simulink model "SortierAlgorithmusVirtuell"  (R2018b)
settings: Solver=FixedStepDiscrete  StartTime=0.0  StopTime=120  RelTol=1e-3  EnableMultiTasking=on
undefined symbols (not defined in the file): sigbuilder_block
libraries: simulink x1, realtime_pacer_lib x1
settings Model: ExtModeTrigDuration=8  Creator=Nici  LastModifiedBy=Nici
settings SolverCC: AutoInsertRateTranBlk=on
settings OptimizationCC: DefaultUnderspecifiedDataType=single  EnhancedBackFolding=on  PassReuseOutputArgsAs=Individual arguments  MaxStackSize=512  OptimizeBlockOrder=speed  DifferentSizesBufferReuse=on  OptimizationCustomize=off
settings DebuggingCC: ParameterTunabilityLossMsg=error  UnderSpecifiedDataTypeMsg=warning
settings HardwareCC: ProdBitPerChar=16  ProdBitPerInt=16  ProdBitPerPointer=32  ProdBitPerSizeT=32  ProdBitPerPtrDiffT=32  ProdLargestAtomicInteger=Integer  ProdLargestAtomicFloat=None  ProdWordSize=16  ProdLongLongMode=on  ProdHWDeviceType=Texas Instruments->C2000
settings SFSimCC: MATLABDynamicMemAlloc=off
settings RTWCC: SystemTargetFile=ert.tlc  HardwareBoard=TI Delfino F2833x  TemplateMakefile=ert_default_tmf  GenerateReport=on  Toolchain=Texas Instruments Code Composer Studio (C2000)  IncludeHyperlinkInReport=on  LaunchReport=on  GenerateTraceInfo=on  GenerateTraceReport=on  GenerateTraceReportSl=on  GenerateTraceReportSf=on  GenerateTraceReportEml=on
settings CodeAppCC: ForceParamTrailComments=on  IgnoreCustomStorageClasses=off  OperatorAnnotations=on  SimulinkDataObjDesc=on  SFDataObjDesc=on  InsertBlockDesc=on
settings ERTTargetCC: CodeReplacementLibrary=TI C28x  SupportContinuousTime=on

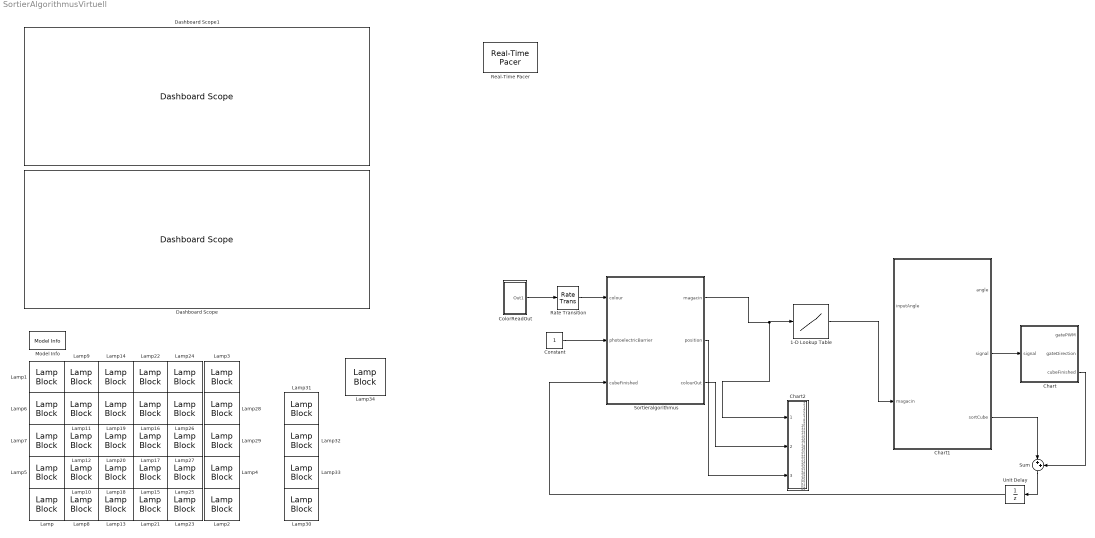
== system SortierAlgorithmusVirtuell ==
  1-D Lookup Table : Lookup_n-D  NumberOfTableDimensions=1  BreakpointsForDimension1=[-1,0,1,2,3,4,5,6]  Table=[-1,-440,-295,-170,-40,85,220,430]  InternalRulePriority=Speed  RndMeth=Simplest  InputSameDT=on
  Chart : Stateflow chart  TreatAsAtomicUnit=on
  Chart1 : Stateflow chart  TreatAsAtomicUnit=on
  Chart2 : Stateflow chart  TreatAsAtomicUnit=on
  ColorReadOut : Subsystem
  Constant : Constant
  Dashboard Scope : DashboardScope  WebBlockId=264  Ymin=-450  Ymax=450
  Dashboard Scope1 : DashboardScope  WebBlockId=268  Ymin=-450  Ymax=450
  Lamp : LampBlock  WebBlockId=196  LabelPosition=Hide
  Lamp1 : LampBlock  WebBlockId=197  LabelPosition=Hide
  Lamp10 : LampBlock  WebBlockId=211  LabelPosition=Hide
  Lamp11 : LampBlock  WebBlockId=212  LabelPosition=Hide
  Lamp12 : LampBlock  WebBlockId=213  LabelPosition=Hide
  Lamp13 : LampBlock  WebBlockId=214  LabelPosition=Hide
  Lamp14 : LampBlock  WebBlockId=215  LabelPosition=Hide
  Lamp15 : LampBlock  WebBlockId=216  LabelPosition=Hide
  Lamp16 : LampBlock  WebBlockId=217  LabelPosition=Hide
  Lamp17 : LampBlock  WebBlockId=218  LabelPosition=Hide
  Lamp18 : LampBlock  WebBlockId=219  LabelPosition=Hide
  Lamp19 : LampBlock  WebBlockId=220  LabelPosition=Hide
  Lamp2 : LampBlock  WebBlockId=249  LabelPosition=Hide
  Lamp20 : LampBlock  WebBlockId=221  LabelPosition=Hide
  Lamp21 : LampBlock  WebBlockId=222  LabelPosition=Hide
  Lamp22 : LampBlock  WebBlockId=223  LabelPosition=Hide
  Lamp23 : LampBlock  WebBlockId=224  LabelPosition=Hide
  Lamp24 : LampBlock  WebBlockId=225  LabelPosition=Hide
  Lamp25 : LampBlock  WebBlockId=226  LabelPosition=Hide
  Lamp26 : LampBlock  WebBlockId=227  LabelPosition=Hide
  Lamp27 : LampBlock  WebBlockId=228  LabelPosition=Hide
  Lamp28 : LampBlock  WebBlockId=252  LabelPosition=Hide
  Lamp29 : LampBlock  WebBlockId=253  LabelPosition=Hide
  Lamp3 : LampBlock  WebBlockId=250  LabelPosition=Hide
  Lamp30 : LampBlock  WebBlockId=257  LabelPosition=Hide
  Lamp31 : LampBlock  WebBlockId=258  LabelPosition=Hide
  Lamp32 : LampBlock  WebBlockId=259  LabelPosition=Hide
  Lamp33 : LampBlock  WebBlockId=260  LabelPosition=Hide
  Lamp34 : LampBlock  WebBlockId=266
  Lamp4 : LampBlock  WebBlockId=251  LabelPosition=Hide
  Lamp5 : LampBlock  WebBlockId=206  LabelPosition=Hide
  Lamp6 : LampBlock  WebBlockId=207  LabelPosition=Hide
  Lamp7 : LampBlock  WebBlockId=208  LabelPosition=Hide
  Lamp8 : LampBlock  WebBlockId=209  LabelPosition=Hide
  Lamp9 : LampBlock  WebBlockId=210  LabelPosition=Hide
  Model Info : simulink/Model-Wide Utilities/Model Info  Frame=on  DisplayStringWithTags=Magazin  HorizontalTextAlignment=Center  LeftAlignmentValue=0.5
  Rate Transition : RateTransition  InitialCondition=1  OutPortSampleTime=0.01
  Real-Time Pacer : realtime_pacer_lib/Real-Time Pacer  simTimePerRealTime=2
  Sortieralgorithmus : Stateflow chart  TreatAsAtomicUnit=on
  Sum : Sum  Inputs=|++
  Unit Delay : UnitDelay  SampleTime=-1
  wires:
  1-D Lookup Table/1 -> Chart1/2(magacin)
  ColorReadOut/1(Out1) -> Rate Transition/1
  Rate Transition/1 -> Sortieralgorithmus/1(colour)
  Chart1/2(signal) -> Chart/1(signal)
  Sortieralgorithmus/1(magacin) -> Chart2/1(magacin), 1-D Lookup Table/1
  Chart/3(cubeFinished) -> Sum/2
  Unit Delay/1 -> Sortieralgorithmus/3(cubeFinished)
  Chart1/3(sortCube) -> Sum/1
  Sum/1 -> Unit Delay/1
  Sortieralgorithmus/2(position) -> Chart2/3(position)
  Sortieralgorithmus/3(colourOut) -> Chart2/2(colour)
  Constant/1 -> Sortieralgorithmus/2(photoelectricBarrier)

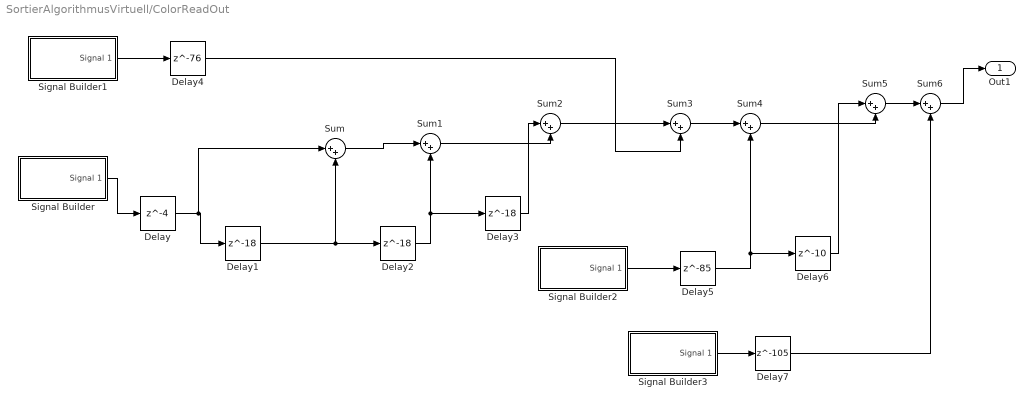
== system SortierAlgorithmusVirtuell/ColorReadOut ==
  Delay : Delay  DelayLength=4  SampleTime=1
  Delay1 : Delay  DelayLength=18  SampleTime=1
  Delay2 : Delay  DelayLength=18  SampleTime=1
  Delay3 : Delay  DelayLength=18  SampleTime=1
  Delay4 : Delay  DelayLength=76  SampleTime=1
  Delay5 : Delay  DelayLength=85  SampleTime=1
  Delay6 : Delay  DelayLength=10  SampleTime=1
  Delay7 : Delay  DelayLength=105  SampleTime=1
  Signal Builder : Subsystem  Tag=STV Subsys  LoadFcn=sigbuilder_block('load');  StartFcn=sigbuilder_block('start');  StopFcn=sigbuilder_block('stop');  ClipboardFcn=sigbuilder_block('clipboard');  mask(Sigbuilder block){tuvar=[0:10]}
      mask help: Simulink:masks:SigbuilderBlock_MD
      mask init:
      | if ~strcmp(get_param(bdroot(gcbh),'SimulationStatus'),'stopped') tuvar = sigbuilder_block('maskInit'); end
      settings: CopyFcn=sigbuilder_block('copy');  DeleteFcn=sigbuilder_block('delete');  ModelCloseFcn=sigbuilder_block('modelClose');  PreSaveFcn=sigbuilder_block('preSave');  PauseFcn=sigbuilder_block('pause');  ContinueFcn=sigbuilder_block('continue');  NameChangeFcn=sigbuilder_block('namechange');  OpenFcn=sigbuilder_block('open',[404.625 154.25 550.5 330.5 ]);  CloseFcn=sigbuilder_block('close');
      mask Display: plot(0, 0, 100, 100,[2, 2, 32, 32, 2], [68, 8, 8, 68, 68],[32, 2], [38, 38], [32, 19, 2],[53, 60, 44], [32, 17, 17, 2],[16, 16, 31, 31]);txt = getActiveGroup(gcbh);text(2, 100, txt,'verticalAlignment', 'top');
  Signal Builder1 : Subsystem  Tag=STV Subsys  LoadFcn=sigbuilder_block('load');  StartFcn=sigbuilder_block('start');  StopFcn=sigbuilder_block('stop');  ClipboardFcn=sigbuilder_block('clipboard');  mask(Sigbuilder block){tuvar=[0:10]}
      mask help: Simulink:masks:SigbuilderBlock_MD
      mask init:
      | if ~strcmp(get_param(bdroot(gcbh),'SimulationStatus'),'stopped') tuvar = sigbuilder_block('maskInit'); end
      settings: CopyFcn=sigbuilder_block('copy');  DeleteFcn=sigbuilder_block('delete');  ModelCloseFcn=sigbuilder_block('modelClose');  PreSaveFcn=sigbuilder_block('preSave');  PauseFcn=sigbuilder_block('pause');  ContinueFcn=sigbuilder_block('continue');  NameChangeFcn=sigbuilder_block('namechange');  OpenFcn=sigbuilder_block('open',[404.625 154.25 550.5 330.5 ]);  CloseFcn=sigbuilder_block('close');
      mask Display: plot(0, 0, 100, 100,[2, 2, 32, 32, 2], [68, 8, 8, 68, 68],[32, 2], [38, 38], [32, 19, 2],[53, 60, 44], [32, 17, 17, 2],[16, 16, 31, 31]);txt = getActiveGroup(gcbh);text(2, 100, txt,'verticalAlignment', 'top');
  Signal Builder2 : Subsystem  Tag=STV Subsys  LoadFcn=sigbuilder_block('load');  StartFcn=sigbuilder_block('start');  StopFcn=sigbuilder_block('stop');  ClipboardFcn=sigbuilder_block('clipboard');  mask(Sigbuilder block){tuvar=[0:10]}
      mask help: Simulink:masks:SigbuilderBlock_MD
      mask init:
      | if ~strcmp(get_param(bdroot(gcbh),'SimulationStatus'),'stopped') tuvar = sigbuilder_block('maskInit'); end
      settings: CopyFcn=sigbuilder_block('copy');  DeleteFcn=sigbuilder_block('delete');  ModelCloseFcn=sigbuilder_block('modelClose');  PreSaveFcn=sigbuilder_block('preSave');  PauseFcn=sigbuilder_block('pause');  ContinueFcn=sigbuilder_block('continue');  NameChangeFcn=sigbuilder_block('namechange');  OpenFcn=sigbuilder_block('open',[190.875 143.25 550.5 330.75 ]);  CloseFcn=sigbuilder_block('close');
      mask Display: plot(0, 0, 100, 100,[2, 2, 32, 32, 2], [68, 8, 8, 68, 68],[32, 2], [38, 38], [32, 19, 2],[53, 60, 44], [32, 17, 17, 2],[16, 16, 31, 31]);txt = getActiveGroup(gcbh);text(2, 100, txt,'verticalAlignment', 'top');
  Signal Builder3 : Subsystem  Tag=STV Subsys  LoadFcn=sigbuilder_block('load');  StartFcn=sigbuilder_block('start');  StopFcn=sigbuilder_block('stop');  ClipboardFcn=sigbuilder_block('clipboard');  mask(Sigbuilder block){tuvar=[0:10]}
      mask help: Simulink:masks:SigbuilderBlock_MD
      mask init:
      | if ~strcmp(get_param(bdroot(gcbh),'SimulationStatus'),'stopped') tuvar = sigbuilder_block('maskInit'); end
      settings: CopyFcn=sigbuilder_block('copy');  DeleteFcn=sigbuilder_block('delete');  ModelCloseFcn=sigbuilder_block('modelClose');  PreSaveFcn=sigbuilder_block('preSave');  PauseFcn=sigbuilder_block('pause');  ContinueFcn=sigbuilder_block('continue');  NameChangeFcn=sigbuilder_block('namechange');  OpenFcn=sigbuilder_block('open',[190.875 143.25 550.5 330.75 ]);  CloseFcn=sigbuilder_block('close');
      mask Display: plot(0, 0, 100, 100,[2, 2, 32, 32, 2], [68, 8, 8, 68, 68],[32, 2], [38, 38], [32, 19, 2],[53, 60, 44], [32, 17, 17, 2],[16, 16, 31, 31]);txt = getActiveGroup(gcbh);text(2, 100, txt,'verticalAlignment', 'top');
  Sum{,1..6} (7 alike) : Sum  Inputs=|++
  Out1 : Outport
  wires:
  Delay3/1 -> Sum2/1
  Sum/1 -> Sum1/1
  Signal Builder/1(Signal 1) -> Delay/1
  Sum1/1 -> Sum2/2
  Delay2/1 -> Delay3/1, Sum1/2
  Delay1/1 -> Delay2/1, Sum/2
  Delay/1 -> Sum/1, Delay1/1
  Sum2/1 -> Sum3/1
  Signal Builder1/1(Signal 1) -> Delay4/1
  Delay4/1 -> Sum3/2
  Signal Builder2/1(Signal 1) -> Delay5/1
  Delay5/1 -> Delay6/1, Sum4/2
  Sum3/1 -> Sum4/1
  Delay6/1 -> Sum5/1
  Sum4/1 -> Sum5/2
  Signal Builder3/1(Signal 1) -> Delay7/1
  Sum6/1 -> Out1/1
  Sum5/1 -> Sum6/1
  Delay7/1 -> Sum6/2

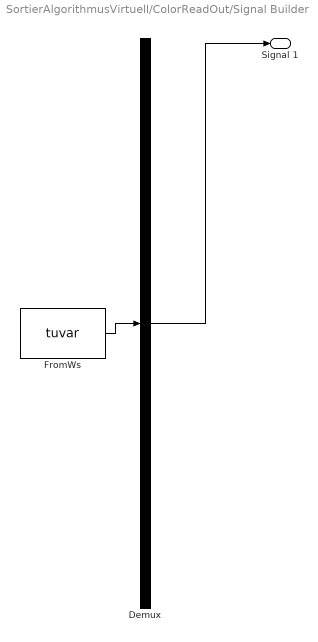
== system SortierAlgorithmusVirtuell/ColorReadOut/Signal Builder ==
  Demux : Demux  Tag=STV Demux  Outputs=1
  FromWs : FromWorkspace  Tag=STV FromWs  VariableName=tuvar  SampleTime=0
      SigBuilderData=|
      | common.afterFinalStr = 'Extrapolate'
      | common.sampleTime = 0
      | dataSet.timeRange = [0 30]
      | dataSet.name = 'Group 1'
      | sbobj.Groups.Name = 'Group 1'
      | sbobj.Groups.Signals.Name = 'Signal 1'
      | sbobj.Groups.Signals.XData = [0 1 1 3 3 4 4 6 6 7 7 9 9 10 10 12 12 13 13 15 15 16 16 21.5 23.3 24.55 25.55 26.7 28.05 30]
      | sbobj.Groups.Signals.YData = [1800 1800 0 0 1800 1800 0 0 2700 2700 0 0 200 200 0 0 1800 1800 0 0 250 250 0 0 0 0 0 0 0 0]
      | sbobj.Groups.TimeRange = [0 30]
  Signal 1 : Outport  Tag=STV Outport
  wires:
  Demux/1 -> Signal 1/1
  FromWs/1 -> Demux/1

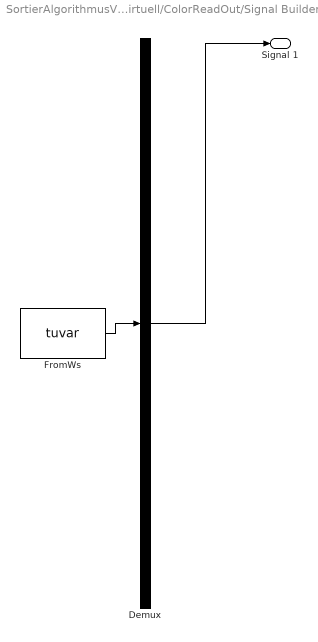
== system SortierAlgorithmusVirtuell/ColorReadOut/Signal Builder1 ==
  Demux : Demux  Tag=STV Demux  Outputs=1
  FromWs : FromWorkspace  Tag=STV FromWs  VariableName=tuvar  SampleTime=0
      SigBuilderData=|
      | common.afterFinalStr = 'Extrapolate'
      | common.sampleTime = 0
      | dataSet.timeRange = [0 30]
      | dataSet.name = 'Group 1'
      | sbobj.Groups.Name = 'Group 1'
      | sbobj.Groups.Signals.Name = 'Signal 1'
      | sbobj.Groups.Signals.XData = [0 1 1 3 3 4 4 6 6 7 7 9 12 21.5 23.3 24.55 25.55 26.7 28.05 30]
      | sbobj.Groups.Signals.YData = [1800 1800 0 0 1800 1800 0 0 250 250 0 0 0 0 0 0 0 0 0 0]
      | sbobj.Groups.TimeRange = [0 30]
  Signal 1 : Outport  Tag=STV Outport
  wires:
  Demux/1 -> Signal 1/1
  FromWs/1 -> Demux/1

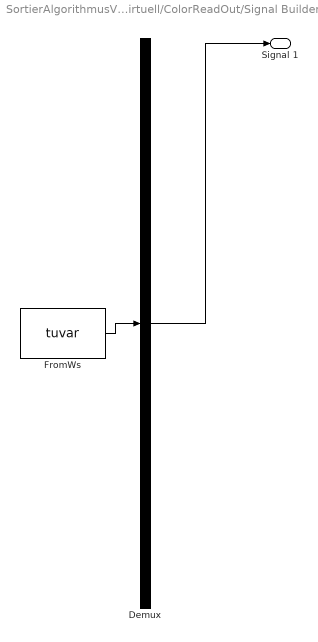
== system SortierAlgorithmusVirtuell/ColorReadOut/Signal Builder2 ==
  Demux : Demux  Tag=STV Demux  Outputs=1
  FromWs : FromWorkspace  Tag=STV FromWs  VariableName=tuvar  SampleTime=0
      SigBuilderData=|
      | common.afterFinalStr = 'Extrapolate'
      | common.sampleTime = 0
      | dataSet.timeRange = [0 30]
      | dataSet.name = 'Group 1'
      | sbobj.Groups.Name = 'Group 1'
      | sbobj.Groups.Signals.Name = 'Signal 1'
      | sbobj.Groups.Signals.XData = [0 1 1 3 3 4 4 6 6 7 7 9 12 21.5 23.3 24.55 25.55 26.7 28.05 30]
      | sbobj.Groups.Signals.YData = [1800 1800 0 0 1800 1800 0 0 1800 1800 0 0 0 0 0 0 0 0 0 0]
      | sbobj.Groups.TimeRange = [0 30]
  Signal 1 : Outport  Tag=STV Outport
  wires:
  Demux/1 -> Signal 1/1
  FromWs/1 -> Demux/1

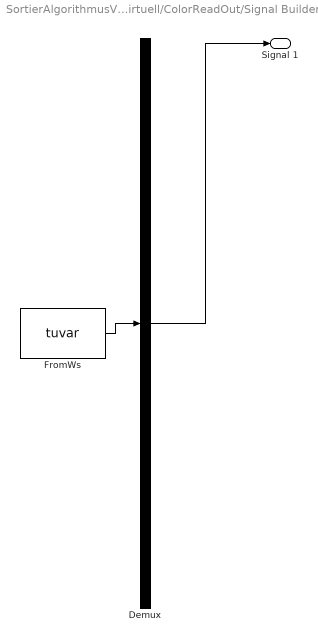
== system SortierAlgorithmusVirtuell/ColorReadOut/Signal Builder3 ==
  Demux : Demux  Tag=STV Demux  Outputs=1
  FromWs : FromWorkspace  Tag=STV FromWs  VariableName=tuvar  SampleTime=0
      SigBuilderData=|
      | common.afterFinalStr = 'Extrapolate'
      | common.sampleTime = 0
      | dataSet.timeRange = [0 30]
      | dataSet.name = 'Group 1'
      | sbobj.Groups.Name = 'Group 1'
      | sbobj.Groups.Signals.Name = 'Signal 1'
      | sbobj.Groups.Signals.XData = [0 1 1 7 9 12 21.5 23.3 24.55 25.55 26.7 28.05 30]
      | sbobj.Groups.Signals.YData = [1800 1800 0 0 0 0 0 0 0 0 0 0 0]
      | sbobj.Groups.TimeRange = [0 30]
  Signal 1 : Outport  Tag=STV Outport
  wires:
  Demux/1 -> Signal 1/1
  FromWs/1 -> Demux/1

== stateflow chart SortierAlgorithmusVirtuell/Chart1 ==
  state firstEntry
    entry: angle = 300;
  note: StartWinkel, da Schieber nicht in Mitte stehen darf am Anfang. 5 Sekunden Zeit um das Bord einzuschalten
  state waitForCube
  state goToZero
    angle = 0;
    sortCube = 1;
  state closeGate
    signal = 0
  state wait
  state openGate
    signal = 1
    sortCube = 0
  state goToMagacin
    entry: angle = magacin;
  (default) -> firstEntry
  firstEntry -> waitForCube : [after(3,sec)]
  closeGate -> waitForCube
  waitForCube -> goToZero : [magacin~= -1]
  goToZero -> wait : [after(1,sec)]
  openGate -> closeGate : [after(0.5, sec)]
  wait -> goToMagacin : [after(0.4, sec)]
  goToMagacin -> openGate : [after(1,sec)]
  data: inputAngle input; magacin input; angle output; signal output; sortCube output single

== stateflow chart SortierAlgorithmusVirtuell/Chart ==
  state wait
    gatePWM = 0
    gateDirection = 1
    cubeFinished = 1
  state close
    gateDirection = 0
  state open
    gatePWM = 50
    cubeFinished = 0
  (default) -> wait
  wait -> open : [signal == 1]
  open -> close : [after(0.3,sec)]
  close -> wait : [after(0.3, sec)]
  data: signal input; gatePWM output; gateDirection output; cubeFinished output

== stateflow chart SortierAlgorithmusVirtuell/Sortieralgorithmus ==
  state setupVariable
    magacin0 = 0;
    magacin1 = 0;
    magacin2 = 0;
    magacin3 = 0;
    magacin4 = 0;
    magacin5 = 0;
    magacin6 = 0;
    magacin0_LastCube = 0;
    magacin1_LastCube = 0;
    magacin2_LastCube = 0;
    magacin3_LastCube = 0;
    magacin4_LastCube = 0;
    magacin5_LastCube = 0;
    magacin6_LastCube = 0;
    magacin = -1;
    blacks = 0;
  state cubeLoaded
    magacin = -1;
  state photoelectricBarrierActivated
  state BlueCube
    entry: magacin = findPlaceForBlue();
    colourOut = 1;
  state RedCube
    entry: magacin = findPlaceForRed();
    colourOut = 2
  state Black
    magacin = 6;
    colourOut = 3;
    position = blacks;
    blacks = blacks + 1;
  state DetectedCube
  setupVariable -> cubeLoaded : [after (3, sec)]
  (default) -> setupVariable
  DetectedCube -> cubeLoaded : [cubeFinished == 0]
  cubeLoaded -> photoelectricBarrierActivated : [photoelectricBarrier < 400]
  photoelectricBarrierActivated -> BlueCube [order 3] : [((colour >= 1000) && (colour <= 2150)) ]
  photoelectricBarrierActivated -> RedCube [order 2] : [(colour < 1000) && (colour > 0)]
  photoelectricBarrierActivated -> Black [order 1] : [(colour > 2150)]
  RedCube -> DetectedCube
  BlueCube -> DetectedCube
  Black -> DetectedCube
  data: magacinOut function_output; magacinOut function_output; colour input; magacin6 local; magacin0_LastCube local; magacin3_LastCube local; magacin2_LastCube local; magacin5_LastCube local; magacin1_LastCube local; magacin6_LastCube local; magacin4_LastCube local; magacin output; photoelectricBarrier input; magacin0 local; magacin1 local; magacin2 local; magacin3 local; magacin4 local; magacin5 local; cubeFinished input; position output; colourOut output; blacks local
  function magacinOut  = findPlaceForRed:
    | function magacinOut  = findPlaceForRed
    | 
    | if((magacin1 == 0) || ((magacin1_LastCube == 1)&& (magacin1 < 5)))
    |             magacinOut = 1;
    |             magacin1 = magacin1 + 1;
    |             magacin1_LastCube = 2;
    |             position = magacin1;
    | elseif (((magacin2_LastCube == 1) && (magacin2 < 5)))
    |             magacinOut = 2;
    |             magacin2 = magacin2 + 1; 
    |             magacin2_LastCube = 2;
    |             position = magacin2;
    | elseif ((magacin0 < 5) && (magacin0 > 0))
    |             magacinOut = 0;
    |             magacin0 = magacin0 + 1;
    |             magacin0_LastCube = 2;
    |             position = magacin0;
    | else 
    |             magacinOut = 3;
    |             magacin3 = magacin3 + 1;
    |             magacin3_LastCube = 2;
    |             position = magacin3;
    | end
  function magacinOut  = findPlaceForBlue:
    | function magacinOut  = findPlaceForBlue
    | 
    | %1 ist Code for Blue, 2 is Code for Red, 3 is Code for Black, 0 is empty
    | if(magacin0 == 0)  
    |             magacinOut = 0;
    |             magacin0 = (magacin0 + 1);
    |             magacin0_LastCube = 1;
    |             position = magacin0;
    | elseif ((magacin2 == 0) || (magacin2_LastCube == 2 && magacin2 < 5))
    |             magacinOut = 2;
    |             magacin2 = magacin2 + 1; 
    |             magacin2_LastCube = 1;
    |             position = magacin2;
    | elseif ((magacin1_LastCube == 2) && (magacin1 < 5))
    |             magacinOut = 1;
    |             magacin1 = magacin1 + 1;
    |             magacin1_LastCube = 1;
    |             position = magacin1;
    | elseif (magacin3 < 5)
    |             magacinOut = 3;
    |             magacin3 = (magacin3 + 1);
    |             position = magacin3;
    | elseif (magacin4 < 5)
    |             magacinOut = 4;
    |             magacin4 = (magacin4 + 1);
    |             position = magacin4;
    | else 
    |             magacinOut = 5;
    |             magacin5 = magacin5 + 1;
    |             position = magacin5;
    | end

== stateflow chart SortierAlgorithmusVirtuell/Chart2 ==
  state Entry
    m11 = 0;
    m12 = 0;
    m13 = 0;
    m14 = 0;
    m15 = 0;
    m21 = 0;
    m22 = 0;
    m23 = 0;
    m24 = 0;
    m25 = 0;
    m31 = 0;
    m32 = 0;
    m33 = 0;
    m34 = 0;
    m35 = 0;
    m41 = 0;
    m42 = 0;
    m43  = 0;
    m44 = 0;
    m45 = 0;
    m51 = 0;
    m52 = 0;
    m53 = 0;
    m54 = 0;
    m55 = 0;
    m61 = 0;
    m62 = 0;
    m63 = 0;
    m64 = 0;
    m65 = 0;
    b1 = 0;
    b2 = 0;
    b3 = 0;
    b0 = 0;
  state Update
    updateColor()
  Entry -> Update
  (default) -> Entry
  data: m11 output; m12 output; m13 output; m14 output; m15 output; magacin input; colour input; position input; m21 output; m22 output; m23 output; m24 output; m25 output; m31 output; m32 output; m33 output; m34 output; m35 output; m41 output; m42 output; m44 output; m45 output; m43 output; m51 output; m52 output; m53 output; m54 output; m55 output; m61 output; m62 output; m63 output; m64 output; m65 output; b0 output; b1 output; b2 output; b3 output
  function updateColor:
    | function updateColor
    | 
    | 
    | 
    | if(magacin == 0)
    |     if(position == 1)
    |         m11 = colour;
    |     elseif(position == 2)
    |         m12 = colour;
    |     elseif(position == 3)
    |         m13 = colour;
    |     elseif(position == 4)
    |         m14 = colour;
    |     elseif(position == 5)
    |         m15 = colour;
    |     end
    | end
    | if(magacin == 1)
    |     if(position == 1)
    |         m21 = colour;
    |     elseif(position == 2)
    |         m22 = colour;
    |     elseif(position == 3)
    |         m23 = colour;
    |     elseif(position == 4)
    |         m24 = colour;
    |     elseif(position == 5)
    |         m25 = colour;
    |     end
    | end
    | if(magacin == 2)
    |     if(position == 1)
    |         m31 = colour;
    |     elseif(position == 2)
    |         m32 = colour;
    |     elseif(position == 3)
    |         m33 = colour;
    |     elseif(position == 4)
    |         m34 = colour;
    |     elseif(position == 5)
    |         m35 = colour;
    |     end
    | 
    | end
    | 
    | if(magacin == 3)
    |     if(position == 1)
    |         m41 = colour;
    |     elseif(position == 2)
    |         m42 = colour;
    |     elseif(position == 3)
    |         m43 = colour;
    |     elseif(position == 4)
    |         m44 = colour;
    |     elseif(position == 5)
    |         m45 = colour;
    |     end
    | 
    | end
    | 
    | if(magacin == 4)
    |     if(position == 1)
    |         m51 = colour;
    |     elseif(position == 2)
    |         m52 = colour;
    |     elseif(position == 3)
    |         m53 = colour;
    |     elseif(position == 4)
    |         m54 = colour;
    |     elseif(position == 5)
    |         m55 = colour;
    |     end
    | 
    | end
    | 
    | if(magacin == 5)
    |     if(position == 1)
    |         m61 = colour;
    |     elseif(position == 2)
    |         m62 = colour;
    |     elseif(position == 3)
    |         m63 = colour;
    |     elseif(position == 4)
    |         m64 = colour;
    |     elseif(position == 5)
    |         m65 = colour;
    |     end
    | end
    | 
    | if(colour == 3)
    |     if(position == 0)
    |         b0 = 1;
    |     elseif(position == 1)
    |         b1 = 1;
    |     elseif(position == 2)
    |         b2 = 1;
    |     elseif(position == 3)
    |         b3 = 1;
    |     end
    | end
